simulink library "CAN_lib"  (R2016b)
settings: Solver=VariableStepAuto  StartTime=0.0  StopTime=10.0  RelTol=1e-3
undefined symbols (not defined in the file or in its folder): CAN, fsw_params, MET, orbit_TLE, sim_params
libraries: MET_lib x1, bus_stubs_fsw x1
settings Model: Creator=taylorreynolds  LastModifiedBy=Taylor

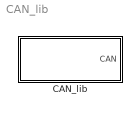
== system CAN_lib ==
  CAN_lib : Subsystem

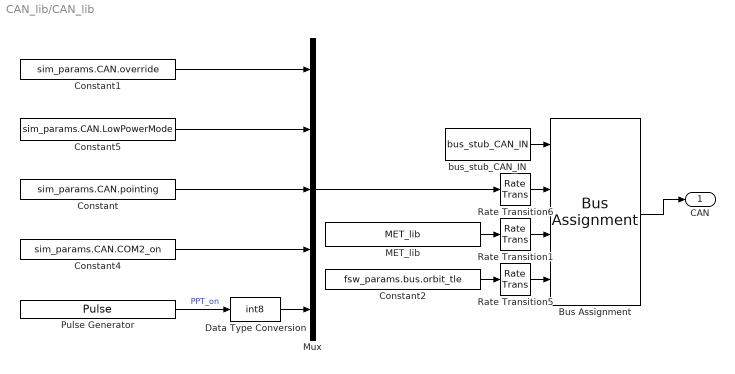
== system CAN_lib/CAN_lib ==
  Bus Assignment : BusAssignment  AssignedSignals=CAN,MET,orbit_TLE
  Constant : Constant  Value=sim_params.CAN.pointing  OutDataTypeStr=int8
  Constant1 : Constant  Value=sim_params.CAN.override  OutDataTypeStr=int8
  Constant2 : Constant  Value=fsw_params.bus.orbit_tle
  Constant4 : Constant  Value=sim_params.CAN.COM2_on  OutDataTypeStr=int8
  Constant5 : Constant  Value=sim_params.CAN.LowPowerMode  OutDataTypeStr=int8
  Data Type Conversion : DataTypeConversion  OutDataTypeStr=int8
  MET_lib : MET_lib/MET_lib
  Mux : Mux  Inputs=5
  Pulse Generator : DiscretePulseGenerator  PulseType=Time based  Period=sim_params.CAN.sync_pulse_period_s  PulseWidth=sim_params.CAN.PPT_on_sync_pct
  Rate Transition1 : RateTransition  X0=sim_params.CAN.ic.MET  OutPortSampleTime=sim_params.CAN.sample_time_s
  Rate Transition5 : RateTransition  X0=fsw_params.bus.orbit_tle  OutPortSampleTime=sim_params.CAN.sample_time_s
  Rate Transition6 : RateTransition  X0=sim_params.CAN.ic.all  OutPortSampleTime=sim_params.CAN.sample_time_s
  bus_stub_CAN_IN : bus_stubs_fsw/bus_stub_CAN_IN
  CAN : Outport
  wires:
  Bus Assignment/1 -> CAN/1
  bus_stub_CAN_IN/1 -> Bus Assignment/1
  Mux/1 -> Rate Transition6/1
  Constant1/1 -> Mux/1
  Constant5/1 -> Mux/2
  Constant/1 -> Mux/3
  Constant4/1 -> Mux/4
  Pulse Generator/1 -> Data Type Conversion/1  "PPT_on"
  MET_lib/1 -> Rate Transition1/1
  Constant2/1 -> Rate Transition5/1
  Rate Transition5/1 -> Bus Assignment/4
  Rate Transition6/1 -> Bus Assignment/2
  Rate Transition1/1 -> Bus Assignment/3
  Data Type Conversion/1 -> Mux/5
